simulink model "state_space_simulink_observer_control101"  (R2023b)
settings: Solver=VariableStepAuto  StartTime=0.0  StopTime=endtime  RelTol=1e-3
undefined symbols (not defined in the file or in its folder): A, Aob, B, Bob, C, Cob, D, Dob, K, P, x0
settings Model: Creator=Anthony  LastModifiedBy=Anthony Rossiter
settings DataIOCC: SaveFormat=StructureWithTime  SignalLogging=off
settings ModelReferenceCC: EnableRefExpFcnMdlSchedulingChecks=on

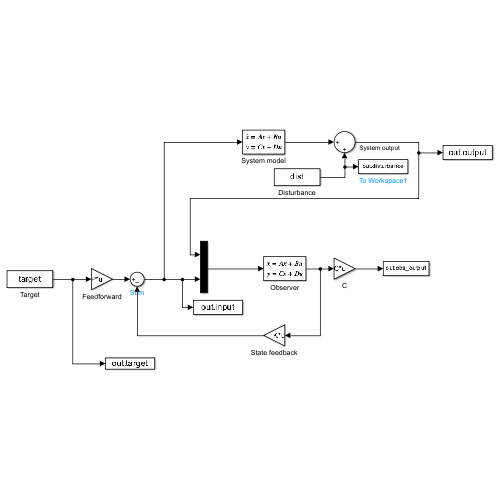
[thumbnail: Simulink's stored preview of the top-level diagram]
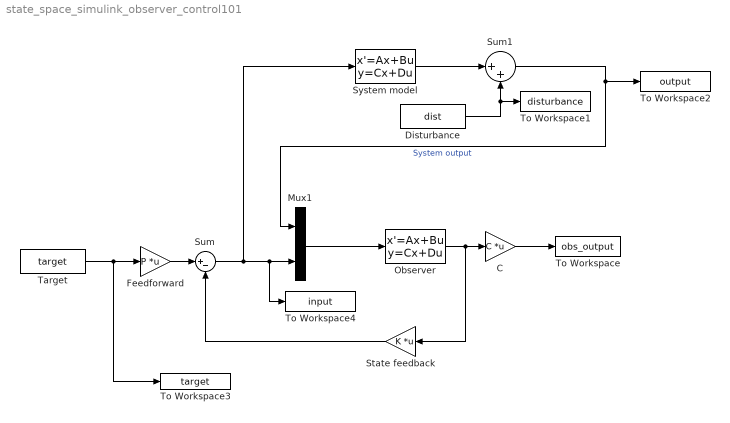
== system state_space_simulink_observer_control101 ==
  C : Gain  Gain=C  Multiplication=Matrix(K*u)
  Disturbance : FromWorkspace  VariableName=dist
  Feedforward : Gain  Gain=P  Multiplication=Matrix(K*u)
  Mux1 : Mux  Inputs=2
  Observer : StateSpace  A=Aob  B=Bob  C=Cob  D=Dob  InitialCondition=0
  State feedback : Gain  Gain=K  Multiplication=Matrix(K*u)
  Sum : Sum  Inputs=|+-
  Sum1 : Sum  Inputs=|++
  System model : StateSpace  A=A  B=B  C=C  D=D  InitialCondition=x0
  Target : FromWorkspace  VariableName=target
  To Workspace : ToWorkspace  VariableName=obs_output  SaveFormat=Structure With Time  SampleTime=-1
  To Workspace1 : ToWorkspace  VariableName=disturbance  SaveFormat=Structure With Time  SampleTime=-1
  To Workspace2 : ToWorkspace  VariableName=output  SaveFormat=Structure With Time  SampleTime=-1
  To Workspace3 : ToWorkspace  VariableName=target  SaveFormat=Structure With Time  SampleTime=-1
  To Workspace4 : ToWorkspace  VariableName=input  SaveFormat=Structure With Time  SampleTime=-1
  wires:
  Observer/1 -> C/1, State feedback/1
  Disturbance/1 -> To Workspace1/1, Sum1/2
  System model/1 -> Sum1/1
  Sum1/1 -> Mux1/1, To Workspace2/1  "System output"
  Feedforward/1 -> Sum/1
  State feedback/1 -> Sum/2
  Sum/1 -> System model/1, To Workspace4/1, Mux1/2
  Mux1/1 -> Observer/1
  Target/1 -> To Workspace3/1, Feedforward/1
  C/1 -> To Workspace/1
